simulink model "sim"  (R2024b)
settings: Solver=VariableStepAuto  StartTime=0.0  StopTime=25  RelTol=1e-3
settings Model: Creator=Ishak  LastModifiedBy=Ishak

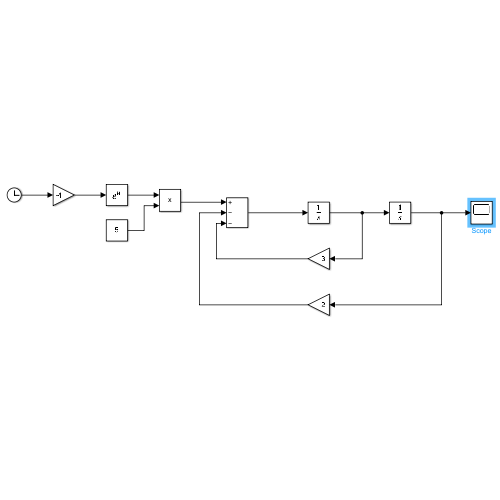
[thumbnail: Simulink's stored preview of the top-level diagram]
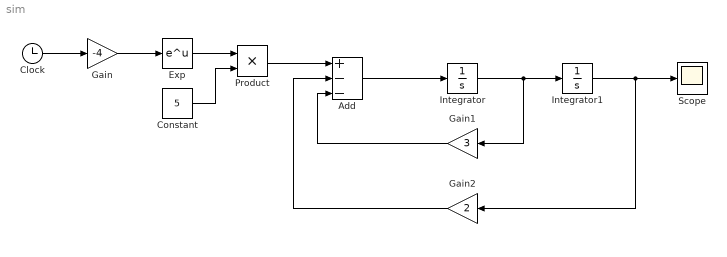
== system sim ==
  Add : Sum  Inputs=+--
  Clock : Clock
  Constant : Constant  Value=5
  Exp : Math
  Gain : Gain  Gain=-4
  Gain1 : Gain  Gain=3
  Gain2 : Gain  Gain=2
  Integrator : Integrator  InitialCondition=-2
  Integrator1 : Integrator  InitialCondition=1
  Product : Product
  Scope : Scope
  wires:
  Add/1 -> Integrator/1
  Integrator/1 -> Gain1/1, Integrator1/1
  Integrator1/1 -> Gain2/1, Scope/1
  Clock/1 -> Gain/1
  Gain/1 -> Exp/1
  Exp/1 -> Product/1
  Constant/1 -> Product/2
  Product/1 -> Add/1
  Gain1/1 -> Add/3
  Gain2/1 -> Add/2
